simulink model "IEEE30_case"  (R2024b)
settings: Solver=FixedStepAuto  StartTime=0  StopTime=5  FixedStep=1e-7  RelTol=1e-3
values from neighbouring files (symbols this model uses):
  GFL_DFIG_7_C_bus = 0.08    [IEEE30_case_parameters.m]
  GFL_DFIG_7_D_mutual = 2.500000e+3    (= 2500)    [IEEE30_case_parameters.m]
  GFL_DFIG_7_f0 = 60    [IEEE30_case_parameters.m]
  GFL_DFIG_7_gPLLi = 3200    [IEEE30_case_parameters.m]
  GFL_DFIG_7_gPLLp = 650    [IEEE30_case_parameters.m]
  GFL_DFIG_7_H_WT = 0.4    [IEEE30_case_parameters.m]
  GFL_DFIG_7_Hg = 0.8    [IEEE30_case_parameters.m]
  GFL_DFIG_7_Igq_ref = 0    [IEEE30_case_parameters.m]
  GFL_DFIG_7_Ird_ref = 704.45696    [IEEE30_case_parameters.m]
  GFL_DFIG_7_KI_V = -300000    [IEEE30_case_parameters.m]
  GFL_DFIG_7_KP_V = -1000    [IEEE30_case_parameters.m]
  GFL_DFIG_7_Ksh = 1.254300e+4    (= 12543)    [IEEE30_case_parameters.m]
  GFL_DFIG_7_Lg = 0.000483    [IEEE30_case_parameters.m]
  GFL_DFIG_7_Lm_pu = 4    [IEEE30_case_parameters.m]
  GFL_DFIG_7_N = 100    [IEEE30_case_parameters.m]
  GFL_DFIG_7_p = 2    [IEEE30_case_parameters.m]
  GFL_DFIG_7_Pitch = 0    [IEEE30_case_parameters.m]
  GFL_DFIG_7_R = 44    [IEEE30_case_parameters.m]
  GFL_DFIG_7_Rg = 2.000000e-5    (= 2e-05)    [IEEE30_case_parameters.m]
  GFL_DFIG_7_rho = 1.225    [IEEE30_case_parameters.m]
  GFL_DFIG_7_rPLLi = 4500    [IEEE30_case_parameters.m]
  GFL_DFIG_7_rPLLp = 620    [IEEE30_case_parameters.m]
  GFL_DFIG_7_Rs_pu = 0.011    [IEEE30_case_parameters.m]
  GFL_DFIG_7_Sbase = 2.000000e+6    (= 2000000)    [IEEE30_case_parameters.m]
  GFL_DFIG_7_ugq_ref = 0    [IEEE30_case_parameters.m]
  GFL_DFIG_7_usd_ref = 0    [IEEE30_case_parameters.m]
  GFL_DFIG_7_Vbase = 690    [IEEE30_case_parameters.m]
  GFL_DFIG_7_Vdc_ref = 1200    [IEEE30_case_parameters.m]
  GFL_DFIG_7_wind = 12    [IEEE30_case_parameters.m]
  GFL_DFIG_7_wm_ref = 518.184209    [IEEE30_case_parameters.m]
  SG_D_13_D = 0.01056    [IEEE30_case_parameters.m]
  SG_D_13_EnableSaturation = 0    [IEEE30_case_parameters.m]
  SG_D_13_f0 = 60    [IEEE30_case_parameters.m]
  SG_D_13_H = 7.5    [IEEE30_case_parameters.m]
  SG_D_13_K_A = 20    [IEEE30_case_parameters.m]
  SG_D_13_K_E = 1.000000e+1    (= 10)    [IEEE30_case_parameters.m]
  SG_D_13_K_F = 2.363    [IEEE30_case_parameters.m]
  SG_D_13_K_s = 0.5    [IEEE30_case_parameters.m]
  SG_D_13_R_a = 0.001088    [IEEE30_case_parameters.m]
  SG_D_13_S_A = 1    [IEEE30_case_parameters.m]
  SG_D_13_S_B = 0.103    [IEEE30_case_parameters.m]
  SG_D_13_S_N = 10.659857    [IEEE30_case_parameters.m]
  SG_D_13_SpeedPara = 200    [IEEE30_case_parameters.m]
  SG_D_13_T_0 = 0.370163    [IEEE30_case_parameters.m]
  SG_D_13_T_1 = 0.3    [IEEE30_case_parameters.m]
  SG_D_13_T_2 = 0.05    [IEEE30_case_parameters.m]
  SG_D_13_T_3 = 0.02    [IEEE30_case_parameters.m]
  SG_D_13_T_4 = 0.005    [IEEE30_case_parameters.m]
  SG_D_13_T_A = 0.02    [IEEE30_case_parameters.m]
  SG_D_13_T_dd = 8.000000e+0    (= 8)    [IEEE30_case_parameters.m]
  SG_D_13_T_ddd = 0.04    [IEEE30_case_parameters.m]
  SG_D_13_T_E = 0.314    [IEEE30_case_parameters.m]
  SG_D_13_T_F = 0.35    [IEEE30_case_parameters.m]
  SG_D_13_T_qd = 0.8    [IEEE30_case_parameters.m]
  SG_D_13_T_qdd = 0.02    [IEEE30_case_parameters.m]
  SG_D_13_T_speed = 0.1    [IEEE30_case_parameters.m]
  SG_D_13_T_w = 0.5    [IEEE30_case_parameters.m]
  SG_D_13_V_ref = 1.696619    [IEEE30_case_parameters.m]
  SG_D_13_w_ref = 376.991118    [IEEE30_case_parameters.m]
  SG_D_13_x_d = 1.9    [IEEE30_case_parameters.m]
  SG_D_13_x_dd = 0.302    [IEEE30_case_parameters.m]
  SG_D_13_x_ddd = 0.204    [IEEE30_case_parameters.m]
  SG_D_13_x_l = 0.05    [IEEE30_case_parameters.m]
  SG_D_13_x_q = 1.3    [IEEE30_case_parameters.m]
  SG_D_13_x_qd = 0.5    [IEEE30_case_parameters.m]
  SG_D_13_x_qdd = 0.3    [IEEE30_case_parameters.m]
  SG_D_1_D = 0.01056    [IEEE30_case_parameters.m]
  SG_D_1_EnableSaturation = 0    [IEEE30_case_parameters.m]
  SG_D_1_f0 = 60    [IEEE30_case_parameters.m]
  SG_D_1_H = 7.5    [IEEE30_case_parameters.m]
  SG_D_1_K_A = 20    [IEEE30_case_parameters.m]
  SG_D_1_K_E = 1.000000e+1    (= 10)    [IEEE30_case_parameters.m]
  SG_D_1_K_F = 2.363    [IEEE30_case_parameters.m]
  SG_D_1_K_s = 0.5    [IEEE30_case_parameters.m]
  SG_D_1_R_a = 0.001088    [IEEE30_case_parameters.m]
  SG_D_1_S_A = 1    [IEEE30_case_parameters.m]
  SG_D_1_S_B = 0.103    [IEEE30_case_parameters.m]
  SG_D_1_S_N = 10.659857    [IEEE30_case_parameters.m]
  SG_D_1_SpeedPara = 200    [IEEE30_case_parameters.m]
  SG_D_1_T_0 = 0.259812    [IEEE30_case_parameters.m]
  SG_D_1_T_1 = 0.3    [IEEE30_case_parameters.m]
  SG_D_1_T_2 = 0.05    [IEEE30_case_parameters.m]
  SG_D_1_T_3 = 0.02    [IEEE30_case_parameters.m]
  SG_D_1_T_4 = 0.005    [IEEE30_case_parameters.m]
  SG_D_1_T_A = 0.02    [IEEE30_case_parameters.m]
  SG_D_1_T_dd = 8.000000e+0    (= 8)    [IEEE30_case_parameters.m]
  SG_D_1_T_ddd = 0.04    [IEEE30_case_parameters.m]
  SG_D_1_T_E = 0.314    [IEEE30_case_parameters.m]
  SG_D_1_T_F = 0.35    [IEEE30_case_parameters.m]
  SG_D_1_T_qd = 0.8    [IEEE30_case_parameters.m]
  SG_D_1_T_qdd = 0.02    [IEEE30_case_parameters.m]
  SG_D_1_T_speed = 0.1    [IEEE30_case_parameters.m]
  SG_D_1_T_w = 0.5    [IEEE30_case_parameters.m]
  SG_D_1_V_ref = 1.544107    [IEEE30_case_parameters.m]
  SG_D_1_w_ref = 376.991118    [IEEE30_case_parameters.m]
  SG_D_1_x_d = 1.9    [IEEE30_case_parameters.m]
  SG_D_1_x_dd = 0.302    [IEEE30_case_parameters.m]
  SG_D_1_x_ddd = 0.204    [IEEE30_case_parameters.m]
  SG_D_1_x_l = 0.05    [IEEE30_case_parameters.m]
  SG_D_1_x_q = 1.3    [IEEE30_case_parameters.m]
  SG_D_1_x_qd = 0.5    [IEEE30_case_parameters.m]
  SG_D_1_x_qdd = 0.3    [IEEE30_case_parameters.m]
  SG_D_22_D = 0.01056    [IEEE30_case_parameters.m]
  SG_D_22_EnableSaturation = 0    [IEEE30_case_parameters.m]
  SG_D_22_f0 = 60    [IEEE30_case_parameters.m]
  SG_D_22_H = 7.5    [IEEE30_case_parameters.m]
  SG_D_22_K_A = 20    [IEEE30_case_parameters.m]
  SG_D_22_K_E = 1.000000e+1    (= 10)    [IEEE30_case_parameters.m]
  SG_D_22_K_F = 2.363    [IEEE30_case_parameters.m]
  SG_D_22_K_s = 0.5    [IEEE30_case_parameters.m]
  SG_D_22_R_a = 0.001088    [IEEE30_case_parameters.m]
  SG_D_22_S_A = 1    [IEEE30_case_parameters.m]
  SG_D_22_S_B = 0.103    [IEEE30_case_parameters.m]
  SG_D_22_S_N = 10.659857    [IEEE30_case_parameters.m]
  SG_D_22_SpeedPara = 200    [IEEE30_case_parameters.m]
  SG_D_22_T_0 = 0.216121    [IEEE30_case_parameters.m]
  SG_D_22_T_1 = 0.3    [IEEE30_case_parameters.m]
  SG_D_22_T_2 = 0.05    [IEEE30_case_parameters.m]
  SG_D_22_T_3 = 0.02    [IEEE30_case_parameters.m]
  SG_D_22_T_4 = 0.005    [IEEE30_case_parameters.m]
  ... (+126 more)
(part 20 of 27)

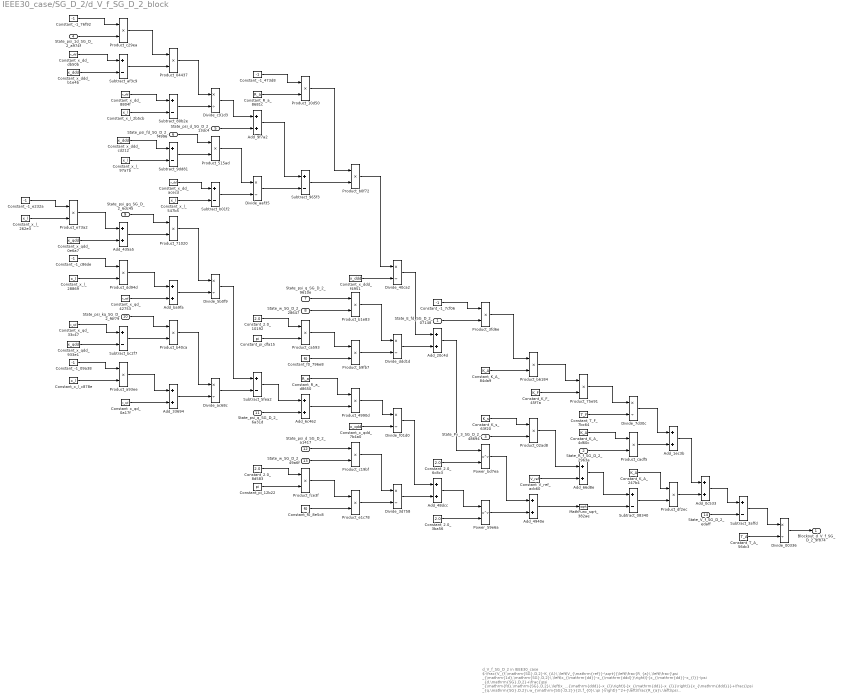
== system IEEE30_case/SG_D_2/d_V_f_SG_D_2_block ==
  note: d_V_f_SG_D_2 in IEEE30_case
      | $-\frac{V_{f,\mathrm{SG},D,2}-K_{A}\,\left(V_{\mathrm{ref}}-\sqrt{{\left(\frac{R_{a}\,\left(\frac{\psi _{\mathrm{1d},\mathrm{SG},D,2}\,\left(x_{\mathrm{dd}}-x_{\mathrm{ddd}}\right)}{x_{\mathrm{dd}}-x_{l}}-\psi _{d,\mathrm{SG},D,2}+\frac{\psi _{\mathrm{fd},\mathrm{SG},D,2}\,\left(x_{\mathrm{ddd}}-x_{l}\right)}{x_{\mathrm{dd}}-x_{l}}\right)}{x_{\mathrm{ddd}}}+\frac{\psi _{q,\mathrm{SG},D,2}\,w_{\mathrm{SG},D,2}}{2\,f_{0}\,\pi }\right)}^2+{\left(\frac{R_{a}\,\left(\psi _{q,\mathrm{SG},D,2}+\frac{\psi _{\mathrm{gq},\mathrm{SG},D,2}\,\left(x_{l}-x_{\mathrm{qdd}}\right)}{x_{l}-x_{\mathrm{qd}}}+\frac{\psi _{\mathrm{kq},\mathrm{SG},D,2}\,\left(x_{\mathrm{qd}}-x_{\mathrm{qdd}}\right)}{x_{l}-x_{\mathrm{qd}}}\right)}{x_{\mathrm{qdd}}}+\frac{\psi _{d,\mathrm{SG},D,2}\,w_{\mathrm{SG},D,2}}{2\,f_{0}\,\pi }\right)}^2}+K_{s}\,\mathrm{Px}_{3,\mathrm{SG},D,2}\right)-K_{A}\,R_{f,\mathrm{SG},D,2}+\frac{E_{\mathrm{fd},\mathrm{SG},D,2}\,K_{A}\,K_{F}}{T_{F}}}{T_{A}}$
      | Automatically generated on 2025-11-01 18:31:41 .
  State_E_fd_SG_D_2_07148 : Inport
  State_R_f_SG_D_2_2963a : Inport  Port=2
  State_Px_3_SG_D_2_48694 : Inport  Port=3
  State_psi_1d_SG_D_2_a974f : Inport  Port=4
  State_psi_d_SG_D_2_13dc4 : Inport  Port=5
  State_psi_fd_SG_D_2_f4996 : Inport  Port=6
  State_psi_q_SG_D_2_9610e : Inport  Port=7
  State_w_SG_D_2_28647 : Inport  Port=8
  State_psi_gq_SG_D_2_6dc45 : Inport  Port=9
  State_psi_kq_SG_D_2_f6f79 : Inport  Port=10
  State_psi_q_SG_D_2_6a31d : Inport  Port=11
  State_psi_d_SG_D_2_a1417 : Inport  Port=12
  State_w_SG_D_2_49a6f : Inport  Port=13
  State_V_f_SG_D_2_edaff : Inport  Port=14
  Add_0c533 : Sum
  Add_1ec3b : Sum
  Add_20c4d : Sum
  Add_33694 : Sum
  Add_435a5 : Sum
  Add_48dcc : Sum
  Add_4940e : Sum
  Add_66d8e : Sum
  Add_6c462 : Sum
  Add_9f7a2 : Sum
  Add_ba9fa : Sum
  Constant_-1_09a38 : Constant  Value=-1
  Constant_-1_473d8 : Constant  Value=-1
  Constant_-1_76f92 : Constant  Value=-1
  Constant_-1_7cf06 : Constant  Value=-1
  Constant_-1_c86de : Constant  Value=-1
  Constant_-1_e232a : Constant  Value=-1
  Constant_2.0_10192 : Constant  Value=2.0
  Constant_2.0_3ba56 : Constant  Value=2.0
  Constant_2.0_6c8c3 : Constant  Value=2.0
  Constant_2.0_8d583 : Constant  Value=2.0
  Constant_K_A_247b4 : Constant  Value=K_A
  Constant_K_A_4d60c : Constant  Value=K_A
  Constant_K_A_84da9 : Constant  Value=K_A
  Constant_K_F_45f7a : Constant  Value=K_F
  Constant_K_s_63f20 : Constant  Value=K_s
  Constant_R_a_8681c : Constant  Value=R_a
  Constant_R_a_d8650 : Constant  Value=R_a
  Constant_T_A_56dc3 : Constant  Value=T_A
  Constant_T_F_7bc64 : Constant  Value=T_F
  Constant_V_ref_acb60 : Constant  Value=V_ref
  Constant_f0_796e8 : Constant  Value=f0
  Constant_f0_8e5c8 : Constant  Value=f0
  Constant_pi_12b22 : Constant  Value=pi
  Constant_pi_dfa15 : Constant  Value=pi
  Constant_x_dd_8804f : Constant  Value=x_dd
  Constant_x_dd_acecd : Constant  Value=x_dd
  Constant_x_dd_db50b : Constant  Value=x_dd
  Constant_x_ddd_b1e4b : Constant  Value=x_ddd
  Constant_x_ddd_cd212 : Constant  Value=x_ddd
  Constant_x_ddd_f4951 : Constant  Value=x_ddd
  Constant_x_l_262e3 : Constant  Value=x_l
  Constant_x_l_28869 : Constant  Value=x_l
  Constant_x_l_2b5cb : Constant  Value=x_l
  Constant_x_l_547b5 : Constant  Value=x_l
  Constant_x_l_97a7b : Constant  Value=x_l
  Constant_x_l_c878e : Constant  Value=x_l
  Constant_x_qd_0a17f : Constant  Value=x_qd
  Constant_x_qd_33c47 : Constant  Value=x_qd
  Constant_x_qd_42753 : Constant  Value=x_qd
  Constant_x_qdd_0e6a7 : Constant  Value=x_qdd
  Constant_x_qdd_7b4a0 : Constant  Value=x_qdd
  Constant_x_qdd_933e1 : Constant  Value=x_qdd
  Divide_00336 : Product  Inputs=*/
  Divide_3d758 : Product  Inputs=*/
  Divide_40ca2 : Product  Inputs=*/
  Divide_5b0f9 : Product  Inputs=*/
  Divide_7d30c : Product  Inputs=*/
  Divide_aaf35 : Product  Inputs=*/
  Divide_ac68c : Product  Inputs=*/
  Divide_c91d3 : Product  Inputs=*/
  Divide_ddd1d : Product  Inputs=*/
  Divide_f01d0 : Product  Inputs=*/
  MathFunc_sqrt_382ae : Sqrt
  Power_59e6a : Math  Operator=pow
  Power_bd7ea : Math  Operator=pow
  Product_02ad8 : Product
  Product_04437 : Product
  Product_10d50 : Product
  Product_3fd6e : Product
  Product_4990d : Product
  Product_515ad : Product
  Product_71020 : Product
  Product_75e91 : Product
  Product_a93ee : Product
  Product_b0f72 : Product
  Product_b1e83 : Product
  Product_b40ca : Product
  Product_b6184 : Product
  Product_b9fb7 : Product
  Product_c19bf : Product
  Product_c29ea : Product
  Product_ca593 : Product
  Product_cadf5 : Product
  Product_dd94d : Product
  Product_df2ec : Product
  Product_e1c78 : Product
  Product_e73a2 : Product
  Product_fce3f : Product
  Subtract_08340 : Sum  Inputs=+-
  Subtract_3affd : Sum  Inputs=+-
  Subtract_5fea2 : Sum  Inputs=+-
  Subtract_80b2e : Sum  Inputs=+-
  Subtract_965f3 : Sum  Inputs=+-
  Subtract_9dd81 : Sum  Inputs=+-
  Subtract_af3c9 : Sum  Inputs=+-
  Subtract_b01f2 : Sum  Inputs=+-
  Subtract_bc2f7 : Sum  Inputs=+-
  Blockout_d_V_f_SG_D_2_9f874 : Outport
  wires:
  Constant_-1_76f92/1 -> Product_c29ea/1
  Constant_2.0_10192/1 -> Product_ca593/1
  Constant_-1_e232a/1 -> Product_e73a2/1
  Product_ca593/1 -> Product_b9fb7/1
  Product_e73a2/1 -> Add_435a5/1
  Constant_x_l_c878e/1 -> Product_a93ee/2
  Constant_x_l_262e3/1 -> Product_e73a2/2
  State_psi_1d_SG_D_2_a974f/1 -> Product_c29ea/2
  Constant_x_l_547b5/1 -> Subtract_b01f2/2
  Constant_x_dd_db50b/1 -> Subtract_af3c9/1
  Product_4990d/1 -> Divide_f01d0/1
  Constant_x_ddd_b1e4b/1 -> Subtract_af3c9/2
  Constant_x_qd_0a17f/1 -> Add_33694/2
  Add_435a5/1 -> Product_71020/2
  Constant_x_qdd_0e6a7/1 -> Add_435a5/2
  Constant_-1_c86de/1 -> Product_dd94d/1
  Constant_x_dd_acecd/1 -> Subtract_b01f2/1
  Subtract_5fea2/1 -> Add_6c462/1
  Power_bd7ea/1 -> Add_4940e/1
  Constant_x_l_28869/1 -> Product_dd94d/2
  Constant_2.0_8d583/1 -> Product_fce3f/1
  Constant_x_qd_33c47/1 -> Subtract_bc2f7/1
  Constant_pi_12b22/1 -> Product_fce3f/2
  Subtract_965f3/1 -> Product_b0f72/2
  Constant_x_qdd_933e1/1 -> Subtract_bc2f7/2
  State_psi_fd_SG_D_2_f4996/1 -> Product_515ad/1
  Constant_-1_09a38/1 -> Product_a93ee/1
  Product_c29ea/1 -> Product_04437/1
  State_w_SG_D_2_49a6f/1 -> Product_c19bf/2
  Subtract_af3c9/1 -> Product_04437/2
  Constant_x_dd_8804f/1 -> Subtract_80b2e/1
  State_psi_q_SG_D_2_6a31d/1 -> Add_6c462/2
  State_w_SG_D_2_28647/1 -> Product_b1e83/2
  Subtract_9dd81/1 -> Product_515ad/2
  Constant_x_l_2b5cb/1 -> Subtract_80b2e/2
  Add_1ec3b/1 -> Add_0c533/1
  Constant_x_ddd_cd212/1 -> Subtract_9dd81/1
  Constant_x_l_97a7b/1 -> Subtract_9dd81/2
  State_psi_gq_SG_D_2_6dc45/1 -> Product_71020/1
  Product_dd94d/1 -> Add_ba9fa/1
  Subtract_b01f2/1 -> Divide_aaf35/2
  Constant_x_qd_42753/1 -> Add_ba9fa/2
  Product_b1e83/1 -> Divide_ddd1d/1
  State_psi_kq_SG_D_2_f6f79/1 -> Product_b40ca/1
  Subtract_bc2f7/1 -> Product_b40ca/2
  Product_515ad/1 -> Divide_aaf35/1
  State_V_f_SG_D_2_edaff/1 -> Subtract_3affd/2
  Product_a93ee/1 -> Add_33694/1
  Product_04437/1 -> Divide_c91d3/1
  Divide_5b0f9/1 -> Subtract_5fea2/1
  Subtract_80b2e/1 -> Divide_c91d3/2
  Product_71020/1 -> Divide_5b0f9/1
  Add_ba9fa/1 -> Divide_5b0f9/2
  Product_b40ca/1 -> Divide_ac68c/1
  Divide_aaf35/1 -> Subtract_965f3/2
  Constant_f0_796e8/1 -> Product_b9fb7/2
  Add_33694/1 -> Divide_ac68c/2
  Divide_c91d3/1 -> Add_9f7a2/1
  State_psi_d_SG_D_2_13dc4/1 -> Add_9f7a2/2
  Divide_ac68c/1 -> Subtract_5fea2/2
  Constant_-1_473d8/1 -> Product_10d50/1
  Constant_R_a_8681c/1 -> Product_10d50/2
  Constant_f0_8e5c8/1 -> Product_e1c78/2
  Add_9f7a2/1 -> Subtract_965f3/1
  Product_10d50/1 -> Product_b0f72/1
  Constant_pi_dfa15/1 -> Product_ca593/2
  State_psi_q_SG_D_2_9610e/1 -> Product_b1e83/1
  Constant_R_a_d8650/1 -> Product_4990d/1
  State_E_fd_SG_D_2_07148/1 -> Product_3fd6e/2
  Add_6c462/1 -> Product_4990d/2
  State_psi_d_SG_D_2_a1417/1 -> Product_c19bf/1
  Product_fce3f/1 -> Product_e1c78/1
  Product_b0f72/1 -> Divide_40ca2/1
  Constant_x_ddd_f4951/1 -> Divide_40ca2/2
  Product_b9fb7/1 -> Divide_ddd1d/2
  Constant_x_qdd_7b4a0/1 -> Divide_f01d0/2
  Product_c19bf/1 -> Divide_3d758/1
  Product_e1c78/1 -> Divide_3d758/2
  Divide_40ca2/1 -> Add_20c4d/1
  Divide_ddd1d/1 -> Add_20c4d/2
  Divide_f01d0/1 -> Add_48dcc/1
  Divide_3d758/1 -> Add_48dcc/2
  Constant_-1_7cf06/1 -> Product_3fd6e/1
  Add_20c4d/1 -> Power_bd7ea/1
  Constant_2.0_6c8c3/1 -> Power_bd7ea/2
  Add_48dcc/1 -> Power_59e6a/1
  Constant_2.0_3ba56/1 -> Power_59e6a/2
  Product_3fd6e/1 -> Product_b6184/1
  Constant_K_A_84da9/1 -> Product_b6184/2
  Constant_K_s_63f20/1 -> Product_02ad8/1
  State_Px_3_SG_D_2_48694/1 -> Product_02ad8/2
  Power_59e6a/1 -> Add_4940e/2
  Product_b6184/1 -> Product_75e91/1
  Constant_K_F_45f7a/1 -> Product_75e91/2
  Product_02ad8/1 -> Add_66d8e/1
  Constant_V_ref_acb60/1 -> Add_66d8e/2
  Add_4940e/1 -> MathFunc_sqrt_382ae/1
  Product_75e91/1 -> Divide_7d30c/1
  Constant_T_F_7bc64/1 -> Divide_7d30c/2
  Constant_K_A_4d60c/1 -> Product_cadf5/1
  State_R_f_SG_D_2_2963a/1 -> Product_cadf5/2
  Add_66d8e/1 -> Subtract_08340/1
  MathFunc_sqrt_382ae/1 -> Subtract_08340/2
  Divide_7d30c/1 -> Add_1ec3b/1
  Product_cadf5/1 -> Add_1ec3b/2
  Constant_K_A_247b4/1 -> Product_df2ec/1
  Subtract_08340/1 -> Product_df2ec/2
  Product_df2ec/1 -> Add_0c533/2
  Add_0c533/1 -> Subtract_3affd/1
  Subtract_3affd/1 -> Divide_00336/1
  Constant_T_A_56dc3/1 -> Divide_00336/2
  Divide_00336/1 -> Blockout_d_V_f_SG_D_2_9f874/1

== system IEEE30_case/SG_D_2/d_psi_1d_SG_D_2_block ==
  note: d_psi_1d_SG_D_2 in IEEE30_case
      | $-\frac{\psi _{\mathrm{1d},\mathrm{SG},D,2}-\psi _{\mathrm{fd},\mathrm{SG},D,2}+\frac{\left(x_{\mathrm{dd}}-x_{l}\right)\,\left(\frac{\psi _{\mathrm{1d},\mathrm{SG},D,2}\,\left(x_{\mathrm{dd}}-x_{\mathrm{ddd}}\right)}{x_{\mathrm{dd}}-x_{l}}-\psi _{d,\mathrm{SG},D,2}+\frac{\psi _{\mathrm{fd},\mathrm{SG},D,2}\,\left(x_{\mathrm{ddd}}-x_{l}\right)}{x_{\mathrm{dd}}-x_{l}}\right)}{x_{\mathrm{ddd}}}}{T_{\mathrm{ddd}}}$
      | Automatically generated on 2025-11-01 18:31:17 .
  State_psi_1d_SG_D_2_46e59 : Inport
  State_psi_fd_SG_D_2_4eec5 : Inport  Port=2
  State_psi_1d_SG_D_2_ea3e5 : Inport  Port=3
  State_psi_d_SG_D_2_140c5 : Inport  Port=4
  State_psi_fd_SG_D_2_f6724 : Inport  Port=5
  Add_553a5 : Sum
  Add_8b957 : Sum
  Add_a40bf : Sum
  Constant_-1_36965 : Constant  Value=-1
  Constant_-1_77d61 : Constant  Value=-1
  Constant_T_ddd_11beb : Constant  Value=T_ddd
  Constant_x_dd_1d866 : Constant  Value=x_dd
  Constant_x_dd_46c81 : Constant  Value=x_dd
  Constant_x_dd_4adc0 : Constant  Value=x_dd
  Constant_x_dd_868cb : Constant  Value=x_dd
  Constant_x_ddd_81e13 : Constant  Value=x_ddd
  Constant_x_ddd_8ebd4 : Constant  Value=x_ddd
  Constant_x_ddd_f80a5 : Constant  Value=x_ddd
  Constant_x_l_73925 : Constant  Value=x_l
  Constant_x_l_aa17b : Constant  Value=x_l
  Constant_x_l_cdd04 : Constant  Value=x_l
  Constant_x_l_d246a : Constant  Value=x_l
  Divide_32af8 : Product  Inputs=*/
  Divide_42413 : Product  Inputs=*/
  Divide_64a93 : Product  Inputs=*/
  Divide_c8e3e : Product  Inputs=*/
  Product_0e046 : Product
  Product_23d08 : Product
  Product_618ac : Product
  Product_95b08 : Product
  Product_a66c9 : Product
  Subtract_03fe7 : Sum  Inputs=+-
  Subtract_29157 : Sum  Inputs=+-
  Subtract_63c3a : Sum  Inputs=+-
  Subtract_6d926 : Sum  Inputs=+-
  Subtract_cffb0 : Sum  Inputs=+-
  Subtract_e3072 : Sum  Inputs=+-
  Blockout_d_psi_1d_SG_D_2_b4ac5 : Outport
  wires:
  Subtract_e3072/1 -> Product_23d08/2
  Constant_x_l_aa17b/1 -> Subtract_03fe7/2
  Divide_32af8/1 -> Add_553a5/2
  Subtract_cffb0/1 -> Product_0e046/2
  Constant_-1_36965/1 -> Product_618ac/1
  Constant_x_dd_4adc0/1 -> Subtract_63c3a/1
  Divide_42413/1 -> Blockout_d_psi_1d_SG_D_2_b4ac5/1
  State_psi_fd_SG_D_2_4eec5/1 -> Add_a40bf/2
  State_psi_1d_SG_D_2_ea3e5/1 -> Product_618ac/2
  Divide_64a93/1 -> Subtract_cffb0/2
  Constant_x_ddd_f80a5/1 -> Subtract_63c3a/2
  State_psi_1d_SG_D_2_46e59/1 -> Product_95b08/2
  Product_618ac/1 -> Product_a66c9/1
  Subtract_63c3a/1 -> Product_a66c9/2
  Constant_x_dd_1d866/1 -> Subtract_03fe7/1
  Constant_x_ddd_8ebd4/1 -> Subtract_e3072/1
  Constant_x_l_73925/1 -> Subtract_e3072/2
  Product_a66c9/1 -> Divide_c8e3e/1
  Subtract_03fe7/1 -> Divide_c8e3e/2
  State_psi_fd_SG_D_2_f6724/1 -> Product_23d08/1
  Constant_x_dd_868cb/1 -> Subtract_6d926/1
  Constant_x_l_cdd04/1 -> Subtract_29157/2
  Constant_x_l_d246a/1 -> Subtract_6d926/2
  Constant_x_ddd_81e13/1 -> Divide_32af8/2
  Divide_c8e3e/1 -> Add_8b957/1
  State_psi_d_SG_D_2_140c5/1 -> Add_8b957/2
  Product_23d08/1 -> Divide_64a93/1
  Subtract_6d926/1 -> Divide_64a93/2
  Constant_x_dd_46c81/1 -> Subtract_29157/1
  Add_8b957/1 -> Subtract_cffb0/1
  Constant_-1_77d61/1 -> Product_95b08/1
  Subtract_29157/1 -> Product_0e046/1
  Product_95b08/1 -> Add_a40bf/1
  Product_0e046/1 -> Divide_32af8/1
  Add_a40bf/1 -> Add_553a5/1
  Add_553a5/1 -> Divide_42413/1
  Constant_T_ddd_11beb/1 -> Divide_42413/2

== system IEEE30_case/SG_D_2/d_psi_d_SG_D_2_block ==
  note: d_psi_d_SG_D_2 in IEEE30_case
      | $2\,\pi \,f_{0}\,\left(v_{d,\mathrm{SG},D,2}\,\sin\left(\theta _{\mathrm{SG},D,2}\right)-v_{q,\mathrm{SG},D,2}\,\cos\left(\theta _{\mathrm{SG},D,2}\right)+\frac{R_{a}\,\left(\frac{\psi _{\mathrm{1d},\mathrm{SG},D,2}\,\left(x_{\mathrm{dd}}-x_{\mathrm{ddd}}\right)}{x_{\mathrm{dd}}-x_{l}}-\psi _{d,\mathrm{SG},D,2}+\frac{\psi _{\mathrm{fd},\mathrm{SG},D,2}\,\left(x_{\mathrm{ddd}}-x_{l}\right)}{x_{\mathrm{dd}}-x_{l}}\right)}{x_{\mathrm{ddd}}}+\frac{\psi _{q,\mathrm{SG},D,2}\,w_{\mathrm{SG},D,2}}{2\,f_{0}\,\pi }\right)$
      | Automatically generated on 2025-11-01 18:31:08 .
  State_psi_1d_SG_D_2_df2dd : Inport
  State_psi_d_SG_D_2_ba6c1 : Inport  Port=2
  State_psi_fd_SG_D_2_fffbd : Inport  Port=3
  Input_v_d_SG_D_2_98b6e : Inport  Port=4
  State_theta_SG_D_2_7fad9 : Inport  Port=5
  Input_v_q_SG_D_2_5c158 : Inport  Port=6
  State_theta_SG_D_2_809cf : Inport  Port=7
  State_psi_q_SG_D_2_54436 : Inport  Port=8
  State_w_SG_D_2_cc748 : Inport  Port=9
  Add_1ebfb : Sum
  Add_63b69 : Sum
  Constant_-1_6ca0d : Constant  Value=-1
  Constant_-2.0_1409b : Constant  Value=-2.0
  Constant_2.0_42c51 : Constant  Value=2.0
  Constant_R_a_27fa6 : Constant  Value=R_a
  Constant_f0_e3338 : Constant  Value=f0
  Constant_f0_fe94e : Constant  Value=f0
  Constant_pi_10ecf : Constant  Value=pi
  Constant_pi_7c0b2 : Constant  Value=pi
  Constant_x_dd_40591 : Constant  Value=x_dd
  Constant_x_dd_65ac5 : Constant  Value=x_dd
  Constant_x_dd_baf94 : Constant  Value=x_dd
  Constant_x_ddd_851e3 : Constant  Value=x_ddd
  Constant_x_ddd_9effc : Constant  Value=x_ddd
  Constant_x_ddd_e26ca : Constant  Value=x_ddd
  Constant_x_l_218e2 : Constant  Value=x_l
  Constant_x_l_5b573 : Constant  Value=x_l
  Constant_x_l_a44df : Constant  Value=x_l
  Divide_3ccb0 : Product  Inputs=*/
  Divide_63f9c : Product  Inputs=*/
  Divide_da75d : Product  Inputs=*/
  Divide_eead1 : Product  Inputs=*/
  MathFunc_cos_24ad6 : Trigonometry  Operator=cos
  MathFunc_sin_91f42 : Trigonometry
  Product_{14361,44426,62010,96773} (4 alike) : Product
  Product_1e194 : Product
  Product_354a5 : Product
  Product_48a05 : Product
  Product_8d88e : Product
  Product_9a8ec : Product
  Product_ae1ce : Product
  Product_ceee8 : Product
  Product_df34b : Product
  Subtract_14ae4 : Sum  Inputs=+-
  Subtract_3cd6b : Sum  Inputs=+-
  Subtract_5791b : Sum  Inputs=+-
  Subtract_85476 : Sum  Inputs=+-
  Subtract_9bf38 : Sum  Inputs=+-
  Subtract_cd5d1 : Sum  Inputs=+-
  Subtract_f9f89 : Sum  Inputs=+-
  Blockout_d_psi_d_SG_D_2_e4800 : Outport
  wires:
  MathFunc_sin_91f42/1 -> Product_df34b/2
  Constant_x_dd_40591/1 -> Subtract_9bf38/1
  Constant_-1_6ca0d/1 -> Product_ae1ce/1
  Constant_x_l_5b573/1 -> Subtract_9bf38/2
  State_psi_1d_SG_D_2_df2dd/1 -> Product_ae1ce/2
  Constant_f0_fe94e/1 -> Product_48a05/2
  Constant_2.0_42c51/1 -> Product_14361/1
  Constant_x_l_218e2/1 -> Subtract_5791b/2
  Constant_x_dd_65ac5/1 -> Subtract_3cd6b/1
  Product_8d88e/1 -> Blockout_d_psi_d_SG_D_2_e4800/1
  Constant_pi_10ecf/1 -> Product_14361/2
  Constant_x_ddd_9effc/1 -> Subtract_3cd6b/2
  Subtract_85476/1 -> Product_8d88e/2
  Product_ae1ce/1 -> Product_9a8ec/1
  Product_14361/1 -> Product_1e194/1
  Subtract_3cd6b/1 -> Product_9a8ec/2
  Divide_eead1/1 -> Subtract_85476/2
  Constant_x_ddd_e26ca/1 -> Subtract_cd5d1/1
  Constant_x_l_a44df/1 -> Subtract_cd5d1/2
  Product_9a8ec/1 -> Divide_3ccb0/1
  Subtract_f9f89/1 -> Add_1ebfb/1
  Subtract_9bf38/1 -> Divide_3ccb0/2
  State_psi_fd_SG_D_2_fffbd/1 -> Product_44426/1
  Subtract_cd5d1/1 -> Product_44426/2
  Constant_x_dd_baf94/1 -> Subtract_5791b/1
  Divide_3ccb0/1 -> Add_63b69/1
  State_psi_d_SG_D_2_ba6c1/1 -> Add_63b69/2
  Product_44426/1 -> Divide_da75d/1
  Subtract_5791b/1 -> Divide_da75d/2
  Add_63b69/1 -> Subtract_14ae4/1
  Divide_da75d/1 -> Subtract_14ae4/2
  Constant_R_a_27fa6/1 -> Product_354a5/1
  Subtract_14ae4/1 -> Product_354a5/2
  Divide_63f9c/1 -> Subtract_f9f89/1
  State_theta_SG_D_2_7fad9/1 -> MathFunc_sin_91f42/1
  Product_354a5/1 -> Divide_63f9c/1
  Constant_-2.0_1409b/1 -> Product_62010/1
  Input_v_d_SG_D_2_98b6e/1 -> Product_df34b/1
  Constant_x_ddd_851e3/1 -> Divide_63f9c/2
  State_theta_SG_D_2_809cf/1 -> MathFunc_cos_24ad6/1
  Product_48a05/1 -> Product_8d88e/1
  Product_df34b/1 -> Subtract_f9f89/2
  Product_62010/1 -> Product_48a05/1
  Input_v_q_SG_D_2_5c158/1 -> Product_ceee8/1
  MathFunc_cos_24ad6/1 -> Product_ceee8/2
  State_psi_q_SG_D_2_54436/1 -> Product_96773/1
  State_w_SG_D_2_cc748/1 -> Product_96773/2
  Constant_f0_e3338/1 -> Product_1e194/2
  Constant_pi_7c0b2/1 -> Product_62010/2
  Product_ceee8/1 -> Add_1ebfb/2
  Product_96773/1 -> Divide_eead1/1
  Product_1e194/1 -> Divide_eead1/2
  Add_1ebfb/1 -> Subtract_85476/1

== system IEEE30_case/SG_D_2/d_psi_fd_SG_D_2_block ==
  note: d_psi_fd_SG_D_2 in IEEE30_case
      | $-\frac{\psi _{\mathrm{fd},\mathrm{SG},D,2}-E_{\mathrm{fd},\mathrm{SG},D,2}+\left(x_{d}-x_{\mathrm{dd}}\right)\,\left(\frac{\frac{\psi _{\mathrm{1d},\mathrm{SG},D,2}\,\left(x_{\mathrm{dd}}-x_{\mathrm{ddd}}\right)}{x_{\mathrm{dd}}-x_{l}}-\psi _{d,\mathrm{SG},D,2}+\frac{\psi _{\mathrm{fd},\mathrm{SG},D,2}\,\left(x_{\mathrm{ddd}}-x_{l}\right)}{x_{\mathrm{dd}}-x_{l}}}{x_{\mathrm{ddd}}}-\frac{\left(x_{\mathrm{dd}}-x_{\mathrm{ddd}}\right)\,\left(\psi _{\mathrm{1d},\mathrm{SG},D,2}-\psi _{\mathrm{fd},\mathrm{SG},D,2}+\frac{\left(x_{\mathrm{dd}}-x_{l}\right)\,\left(\frac{\psi _{\mathrm{1d},\mathrm{SG},D,2}\,\left(x_{\mathrm{dd}}-x_{\mathrm{ddd}}\right)}{x_{\mathrm{dd}}-x_{l}}-\psi _{d,\mathrm{SG},D,2}+\frac{\psi _{\mathrm{fd},\mathrm{SG},D,2}\,\left(x_{\mathrm{ddd}}-x_{l}\right)}{x_{\mathrm{dd}}-x_{l}}\right)}{x_{\mathrm{ddd}}}\right)}{{\left(x_{\mathrm{dd}}-x_{l}\right)}^2}\right)}{T_{\mathrm{dd}}}$
      | Automatically generated on 2025-11-01 18:31:16 .
  State_E_fd_SG_D_2_9e073 : Inport
  State_psi_fd_SG_D_2_a9693 : Inport  Port=2
  State_psi_1d_SG_D_2_36843 : Inport  Port=3
  State_psi_fd_SG_D_2_74282 : Inport  Port=4
  State_psi_1d_SG_D_2_42d8b : Inport  Port=5
  State_psi_d_SG_D_2_4b3f7 : Inport  Port=6
  State_psi_fd_SG_D_2_d0da0 : Inport  Port=7
  State_psi_1d_SG_D_2_a65ff : Inport  Port=8
  State_psi_d_SG_D_2_ea571 : Inport  Port=9
  State_psi_fd_SG_D_2_33a5d : Inport  Port=10
  Add_89e72 : Sum
  Add_bda76 : Sum
  Constant_-1_5d8da : Constant  Value=-1
  Constant_-1_d567e : Constant  Value=-1
  Constant_-1_df985 : Constant  Value=-1
  Constant_2.0_d00af : Constant  Value=2.0
  Constant_T_dd_c33b1 : Constant  Value=T_dd
  Constant_x_d_3bec6 : Constant  Value=x_d
  Constant_x_dd_2654a : Constant  Value=x_dd
  Constant_x_dd_35d89 : Constant  Value=x_dd
  Constant_x_dd_3dab0 : Constant  Value=x_dd
  Constant_x_dd_49b97 : Constant  Value=x_dd
  Constant_x_dd_5107f : Constant  Value=x_dd
  Constant_x_dd_6fcf5 : Constant  Value=x_dd
  Constant_x_dd_b77ee : Constant  Value=x_dd
  Constant_x_dd_ccfa6 : Constant  Value=x_dd
  Constant_x_dd_d0405 : Constant  Value=x_dd
  Constant_x_dd_f5fa7 : Constant  Value=x_dd
  Constant_x_ddd_138bb : Constant  Value=x_ddd
  Constant_x_ddd_2fcd0 : Constant  Value=x_ddd
  Constant_x_ddd_31f43 : Constant  Value=x_ddd
  Constant_x_ddd_38a94 : Constant  Value=x_ddd
  Constant_x_ddd_85702 : Constant  Value=x_ddd
  Constant_x_ddd_be99a : Constant  Value=x_ddd
  Constant_x_ddd_e45f6 : Constant  Value=x_ddd
  Constant_x_l_12728 : Constant  Value=x_l
  Constant_x_l_2384f : Constant  Value=x_l
  Constant_x_l_3369a : Constant  Value=x_l
  Constant_x_l_502c0 : Constant  Value=x_l
  Constant_x_l_8e844 : Constant  Value=x_l
  Constant_x_l_ad53e : Constant  Value=x_l
  Constant_x_l_ba863 : Constant  Value=x_l
  Constant_x_l_c2edc : Constant  Value=x_l
  Divide_12ded : Product  Inputs=*/
  Divide_203f2 : Product  Inputs=*/
  Divide_3c241 : Product  Inputs=*/
  Divide_8473f : Product  Inputs=*/
  Divide_b37b7 : Product  Inputs=*/
  Divide_b90e9 : Product  Inputs=*/
  Divide_f9373 : Product  Inputs=*/
  Divide_fe3e6 : Product  Inputs=*/
  Power_f27f9 : Math  Operator=pow
  Product_19bd0 : Product
  Product_22933 : Product
  Product_53866 : Product
  Product_5c5ca : Product
  Product_7915e : Product
  Product_99b2c : Product
  Product_c0bf3 : Product
  Product_c69e9 : Product
  Product_cdde0 : Product
  Product_f1df4 : Product
  Subtract_04251 : Sum  Inputs=+-
  Subtract_04fdd : Sum  Inputs=+-
  Subtract_07802 : Sum  Inputs=+-
  Subtract_1a333 : Sum  Inputs=+-
  Subtract_1f428 : Sum  Inputs=+-
  Subtract_227c2 : Sum  Inputs=+-
  Subtract_2900f : Sum  Inputs=+-
  Subtract_2c044 : Sum  Inputs=+-
  Subtract_3bae6 : Sum  Inputs=+-
  Subtract_4933a : Sum  Inputs=+-
  Subtract_4a22d : Sum  Inputs=+-
  Subtract_63054 : Sum  Inputs=+-
  Subtract_73adc : Sum  Inputs=+-
  Subtract_7f09d : Sum  Inputs=+-
  Subtract_96f5f : Sum  Inputs=+-
  Subtract_9b979 : Sum  Inputs=+-
  Subtract_9ca98 : Sum  Inputs=+-
  Subtract_bf46b : Sum  Inputs=+-
  Subtract_fe9dc : Sum  Inputs=+-
  Blockout_d_psi_fd_SG_D_2_9f80c : Outport
  wires:
  Constant_x_dd_6fcf5/1 -> Subtract_63054/1
  Constant_-1_5d8da/1 -> Product_cdde0/1
  Constant_x_l_c2edc/1 -> Subtract_07802/2
  Divide_12ded/1 -> Add_bda76/1
  Subtract_04251/1 -> Product_99b2c/2
  Constant_x_l_3369a/1 -> Subtract_63054/2
  Product_99b2c/1 -> Divide_b90e9/1
  State_psi_1d_SG_D_2_42d8b/1 -> Product_cdde0/2
  Constant_x_dd_d0405/1 -> Subtract_73adc/1
  Product_c69e9/1 -> Divide_12ded/1
  Constant_x_dd_49b97/1 -> Subtract_fe9dc/1
  Constant_x_ddd_e45f6/1 -> Subtract_73adc/2
  Constant_x_dd_f5fa7/1 -> Subtract_9ca98/1
  Product_cdde0/1 -> Product_5c5ca/1
  Subtract_73adc/1 -> Product_5c5ca/2
  State_psi_d_SG_D_2_ea571/1 -> Add_bda76/2
  Constant_x_ddd_31f43/1 -> Subtract_04251/1
  Constant_x_l_2384f/1 -> Subtract_04251/2
  Product_5c5ca/1 -> Divide_3c241/1
  Subtract_63054/1 -> Divide_3c241/2
  State_psi_fd_SG_D_2_d0da0/1 -> Product_99b2c/1
  Subtract_2c044/1 -> Product_c0bf3/2
  Constant_x_dd_b77ee/1 -> Subtract_3bae6/1
  Constant_x_l_502c0/1 -> Subtract_3bae6/2
  Product_f1df4/1 -> Product_c0bf3/1
  Divide_3c241/1 -> Add_89e72/1
  State_psi_d_SG_D_2_4b3f7/1 -> Add_89e72/2
  Subtract_3bae6/1 -> Divide_b90e9/2
  Constant_x_dd_2654a/1 -> Subtract_07802/1
  Constant_x_ddd_be99a/1 -> Subtract_2900f/1
  Add_89e72/1 -> Subtract_96f5f/1
  Divide_b90e9/1 -> Subtract_96f5f/2
  Constant_-1_d567e/1 -> Product_19bd0/1
  Product_7915e/1 -> Divide_f9373/1
  State_psi_1d_SG_D_2_a65ff/1 -> Product_19bd0/2
  Subtract_fe9dc/1 -> Product_f1df4/2
  Constant_x_dd_35d89/1 -> Subtract_4a22d/1
  Divide_f9373/1 -> Subtract_9b979/2
  Constant_-1_df985/1 -> Product_f1df4/1
  Constant_x_ddd_138bb/1 -> Subtract_4a22d/2
  Constant_x_ddd_85702/1 -> Divide_203f2/2
  Subtract_07802/1 -> Product_22933/1
  Subtract_96f5f/1 -> Product_22933/2
  State_psi_fd_SG_D_2_74282/1 -> Subtract_227c2/2
  Product_19bd0/1 -> Product_c69e9/1
  Subtract_4a22d/1 -> Product_c69e9/2
  Constant_2.0_d00af/1 -> Power_f27f9/2
  State_psi_1d_SG_D_2_36843/1 -> Subtract_227c2/1
  Constant_x_dd_5107f/1 -> Subtract_04fdd/1
  Subtract_2900f/1 -> Product_7915e/2
  Constant_x_l_12728/1 -> Subtract_04fdd/2
  Constant_x_l_ad53e/1 -> Subtract_2900f/2
  Constant_x_ddd_38a94/1 -> Subtract_fe9dc/2
  Subtract_9ca98/1 -> Divide_f9373/2
  Product_22933/1 -> Divide_203f2/1
  Subtract_04fdd/1 -> Divide_12ded/2
  State_psi_fd_SG_D_2_33a5d/1 -> Product_7915e/1
  Constant_x_l_ba863/1 -> Subtract_9ca98/2
  Constant_x_dd_3dab0/1 -> Subtract_1f428/1
  Subtract_227c2/1 -> Subtract_2c044/1
  Divide_203f2/1 -> Subtract_2c044/2
  Constant_x_l_8e844/1 -> Subtract_1f428/2
  Subtract_1f428/1 -> Power_f27f9/1
  Add_bda76/1 -> Subtract_9b979/1
  Product_c0bf3/1 -> Divide_8473f/1
  Power_f27f9/1 -> Divide_8473f/2
  Subtract_9b979/1 -> Divide_fe3e6/1
  Constant_x_ddd_2fcd0/1 -> Divide_fe3e6/2
  Constant_x_d_3bec6/1 -> Subtract_7f09d/1
  Constant_x_dd_ccfa6/1 -> Subtract_7f09d/2
  Divide_8473f/1 -> Subtract_4933a/1
  Divide_fe3e6/1 -> Subtract_4933a/2
  State_E_fd_SG_D_2_9e073/1 -> Subtract_1a333/1
  State_psi_fd_SG_D_2_a9693/1 -> Subtract_1a333/2
  Subtract_7f09d/1 -> Product_53866/1
  Subtract_4933a/1 -> Product_53866/2
  Subtract_1a333/1 -> Subtract_bf46b/1
  Product_53866/1 -> Subtract_bf46b/2
  Subtract_bf46b/1 -> Divide_b37b7/1
  Constant_T_dd_c33b1/1 -> Divide_b37b7/2
  Divide_b37b7/1 -> Blockout_d_psi_fd_SG_D_2_9f80c/1

== system IEEE30_case/SG_D_2/d_psi_gq_SG_D_2_block ==
  note: d_psi_gq_SG_D_2 in IEEE30_case
      | $-\frac{\psi _{\mathrm{gq},\mathrm{SG},D,2}+\left(x_{q}-x_{\mathrm{qd}}\right)\,\left(\frac{\psi _{q,\mathrm{SG},D,2}+\frac{\psi _{\mathrm{gq},\mathrm{SG},D,2}\,\left(x_{l}-x_{\mathrm{qdd}}\right)}{x_{l}-x_{\mathrm{qd}}}+\frac{\psi _{\mathrm{kq},\mathrm{SG},D,2}\,\left(x_{\mathrm{qd}}-x_{\mathrm{qdd}}\right)}{x_{l}-x_{\mathrm{qd}}}}{x_{\mathrm{qdd}}}+\frac{\left(x_{\mathrm{qd}}-x_{\mathrm{qdd}}\right)\,\left(\psi _{\mathrm{gq},\mathrm{SG},D,2}+\psi _{\mathrm{kq},\mathrm{SG},D,2}+\frac{\left(x_{l}-x_{\mathrm{qd}}\right)\,\left(\psi _{q,\mathrm{SG},D,2}+\frac{\psi _{\mathrm{gq},\mathrm{SG},D,2}\,\left(x_{l}-x_{\mathrm{qdd}}\right)}{x_{l}-x_{\mathrm{qd}}}+\frac{\psi _{\mathrm{kq},\mathrm{SG},D,2}\,\left(x_{\mathrm{qd}}-x_{\mathrm{qdd}}\right)}{x_{l}-x_{\mathrm{qd}}}\right)}{x_{\mathrm{qdd}}}\right)}{{\left(x_{l}-x_{\mathrm{qd}}\right)}^2}\right)}{T_{\mathrm{qd}}}$
      | Automatically generated on 2025-11-01 18:31:22 .
  State_psi_gq_SG_D_2_104a2 : Inport
  State_psi_gq_SG_D_2_afe73 : Inport  Port=2
  State_psi_kq_SG_D_2_5e865 : Inport  Port=3
  State_psi_gq_SG_D_2_1bb75 : Inport  Port=4
  State_psi_kq_SG_D_2_721d7 : Inport  Port=5
  State_psi_q_SG_D_2_83abf : Inport  Port=6
  State_psi_gq_SG_D_2_e51c7 : Inport  Port=7
  State_psi_kq_SG_D_2_7a2a4 : Inport  Port=8
  State_psi_q_SG_D_2_6cd36 : Inport  Port=9
  Add_21c7f : Sum
  Add_2272d : Sum
  Add_3a373 : Sum
  Add_55692 : Sum
  Add_6f089 : Sum
  Add_9a316 : Sum
  Add_c5e13 : Sum
  Add_cff41 : Sum
  Add_d6c76 : Sum
  Add_dab0d : Sum
  Add_f66a3 : Sum
  Add_f8fe5 : Sum
  Constant_-1_10102 : Constant  Value=-1
  Constant_-1_192d4 : Constant  Value=-1
  Constant_-1_290d7 : Constant  Value=-1
  Constant_-1_36899 : Constant  Value=-1
  Constant_-1_3896d : Constant  Value=-1
  Constant_-1_49486 : Constant  Value=-1
  Constant_-1_6c94d : Constant  Value=-1
  Constant_-1_9a49b : Constant  Value=-1
  Constant_-1_c7fce : Constant  Value=-1
  Constant_-1_caba0 : Constant  Value=-1
  Constant_2.0_389d0 : Constant  Value=2.0
  Constant_T_qd_d29d9 : Constant  Value=T_qd
  Constant_x_l_0ae25 : Constant  Value=x_l
  Constant_x_l_12adf : Constant  Value=x_l
  Constant_x_l_1d50c : Constant  Value=x_l
  Constant_x_l_3b729 : Constant  Value=x_l
  Constant_x_l_4b0fb : Constant  Value=x_l
  Constant_x_l_71427 : Constant  Value=x_l
  Constant_x_l_7c493 : Constant  Value=x_l
  Constant_x_l_e27ca : Constant  Value=x_l
  Constant_x_q_d60a7 : Constant  Value=x_q
  Constant_x_qd_2e24b : Constant  Value=x_qd
  Constant_x_qd_30c63 : Constant  Value=x_qd
  Constant_x_qd_320e1 : Constant  Value=x_qd
  Constant_x_qd_3622f : Constant  Value=x_qd
  Constant_x_qd_578ee : Constant  Value=x_qd
  Constant_x_qd_c8aef : Constant  Value=x_qd
  Constant_x_qd_d8f6f : Constant  Value=x_qd
  Constant_x_qd_de86d : Constant  Value=x_qd
  Constant_x_qd_e8870 : Constant  Value=x_qd
  Constant_x_qd_f702b : Constant  Value=x_qd
  Constant_x_qdd_19ca0 : Constant  Value=x_qdd
  Constant_x_qdd_82582 : Constant  Value=x_qdd
  Constant_x_qdd_ac4b7 : Constant  Value=x_qdd
  Constant_x_qdd_b6451 : Constant  Value=x_qdd
  Constant_x_qdd_ba097 : Constant  Value=x_qdd
  Constant_x_qdd_f7649 : Constant  Value=x_qdd
  Constant_x_qdd_fdfde : Constant  Value=x_qdd
  Divide_1c641 : Product  Inputs=*/
  Divide_2a2b0 : Product  Inputs=*/
  Divide_2d9c6 : Product  Inputs=*/
  Divide_2ede0 : Product  Inputs=*/
  Divide_30f9e : Product  Inputs=*/
  Divide_33160 : Product  Inputs=*/
  Divide_60014 : Product  Inputs=*/
  Divide_96e21 : Product  Inputs=*/
  Power_7d008 : Math  Operator=pow
  Product_0c6e7 : Product
  Product_{37177,54883,65103,97917} (4 alike) : Product
  Product_3ed5e : Product
  Product_40b5a : Product
  Product_5283f : Product
  Product_6eed5 : Product
  Product_89c4d : Product
  Product_9a49c : Product
  Product_9d6ad : Product
  Product_b6e50 : Product
  Product_bfbea : Product
  Product_c9315 : Product
  Product_d0ebf : Product
  Product_e22ef : Product
  Subtract_1a0d9 : Sum  Inputs=+-
  Subtract_1ea22 : Sum  Inputs=+-
  Subtract_263b1 : Sum  Inputs=+-
  Subtract_2a63c : Sum  Inputs=+-
  Subtract_4ba7d : Sum  Inputs=+-
  Subtract_9f12a : Sum  Inputs=+-
  Subtract_a0273 : Sum  Inputs=+-
  Subtract_a6d49 : Sum  Inputs=+-
  Blockout_d_psi_gq_SG_D_2_e9d2a : Outport
  wires:
  Constant_x_l_4b0fb/1 -> Product_e22ef/2
  Constant_x_l_3b729/1 -> Product_5283f/2
  Constant_x_qd_de86d/1 -> Subtract_1ea22/1
  Constant_x_l_1d50c/1 -> Product_9d6ad/2
  Constant_x_qdd_ba097/1 -> Subtract_a0273/2
  Constant_-1_10102/1 -> Product_89c4d/1
  Constant_-1_9a49b/1 -> Product_3ed5e/1
  State_psi_gq_SG_D_2_afe73/1 -> Add_3a373/1
  Constant_x_qdd_fdfde/1 -> Subtract_1ea22/2
  Constant_x_qd_e8870/1 -> Subtract_a0273/1
  Constant_x_l_12adf/1 -> Product_89c4d/2
  Constant_x_l_7c493/1 -> Product_3ed5e/2
  Product_89c4d/1 -> Add_dab0d/1
  Product_3ed5e/1 -> Add_2272d/1
  Constant_x_l_71427/1 -> Product_37177/2
  Constant_x_l_0ae25/1 -> Product_0c6e7/2
  Constant_x_qd_f702b/1 -> Add_dab0d/2
  Constant_x_qdd_b6451/1 -> Add_2272d/2
  Constant_-1_c7fce/1 -> Product_37177/1
  Constant_x_qd_3622f/1 -> Add_d6c76/2
  Constant_x_qdd_f7649/1 -> Add_c5e13/2
  State_psi_gq_SG_D_2_1bb75/1 -> Product_d0ebf/1
  Add_dab0d/1 -> Divide_33160/2
  Add_2272d/1 -> Product_d0ebf/2
  Constant_x_qd_320e1/1 -> Subtract_4ba7d/2
  Product_37177/1 -> Add_f66a3/1
  Constant_x_qd_c8aef/1 -> Add_f66a3/2
  State_psi_kq_SG_D_2_721d7/1 -> Product_6eed5/1
  Divide_2a2b0/1 -> Subtract_9f12a/1
  Subtract_1ea22/1 -> Product_6eed5/2
  Product_d0ebf/1 -> Divide_2a2b0/1
  Add_f66a3/1 -> Divide_2a2b0/2
  Add_6f089/1 -> Product_bfbea/2
  Product_6eed5/1 -> Divide_33160/1
  Constant_-1_36899/1 -> Product_0c6e7/1
  Divide_33160/1 -> Subtract_9f12a/2
  Constant_-1_6c94d/1 -> Product_e22ef/1
  Constant_-1_caba0/1 -> Product_5283f/1
  Product_0c6e7/1 -> Add_cff41/1
  Constant_x_qdd_19ca0/1 -> Subtract_1a0d9/2
  Constant_x_qd_d8f6f/1 -> Add_cff41/2
  Subtract_9f12a/1 -> Add_6f089/1
  Constant_-1_192d4/1 -> Product_9d6ad/1
  State_psi_q_SG_D_2_83abf/1 -> Add_6f089/2
  Product_e22ef/1 -> Add_d6c76/1
  Product_5283f/1 -> Add_c5e13/1
  Constant_-1_290d7/1 -> Product_b6e50/1
  Product_bfbea/1 -> Divide_2d9c6/1
  Constant_x_l_e27ca/1 -> Product_b6e50/2
  Product_54883/1 -> Add_9a316/2
  Constant_x_qd_2e24b/1 -> Subtract_1a0d9/1
  Add_cff41/1 -> Product_bfbea/1
  State_psi_gq_SG_D_2_e51c7/1 -> Product_40b5a/1
  Add_d6c76/1 -> Divide_30f9e/2
  Add_c5e13/1 -> Product_40b5a/2
  Product_b6e50/1 -> Add_55692/1
  Constant_x_qd_578ee/1 -> Add_55692/2
  State_psi_kq_SG_D_2_7a2a4/1 -> Product_c9315/1
  Subtract_1a0d9/1 -> Product_c9315/2
  Divide_30f9e/1 -> Subtract_263b1/2
  State_psi_kq_SG_D_2_5e865/1 -> Add_3a373/2
  Product_c9315/1 -> Divide_30f9e/1
  Constant_x_qdd_ac4b7/1 -> Divide_2d9c6/2
  Product_40b5a/1 -> Divide_60014/1
  Add_55692/1 -> Divide_60014/2
  Constant_-1_49486/1 -> Product_97917/1
  Subtract_a0273/1 -> Product_97917/2
  Add_3a373/1 -> Subtract_a6d49/1
  Divide_2d9c6/1 -> Subtract_a6d49/2
  Product_9d6ad/1 -> Add_f8fe5/1
  Constant_x_qd_30c63/1 -> Add_f8fe5/2
  Divide_60014/1 -> Subtract_263b1/1
  Product_97917/1 -> Product_65103/1
  Subtract_a6d49/1 -> Product_65103/2
  Add_f8fe5/1 -> Power_7d008/1
  Constant_2.0_389d0/1 -> Power_7d008/2
  Subtract_263b1/1 -> Add_21c7f/1
  State_psi_q_SG_D_2_6cd36/1 -> Add_21c7f/2
  Product_65103/1 -> Divide_1c641/1
  Power_7d008/1 -> Divide_1c641/2
  Add_21c7f/1 -> Divide_96e21/1
  Constant_x_qdd_82582/1 -> Divide_96e21/2
  Constant_x_q_d60a7/1 -> Subtract_4ba7d/1
  Divide_1c641/1 -> Subtract_2a63c/1
  Divide_96e21/1 -> Subtract_2a63c/2
  Divide_2ede0/1 -> Blockout_d_psi_gq_SG_D_2_e9d2a/1
  Constant_-1_3896d/1 -> Product_9a49c/1
  State_psi_gq_SG_D_2_104a2/1 -> Product_9a49c/2
  Subtract_4ba7d/1 -> Product_54883/1
  Subtract_2a63c/1 -> Product_54883/2
  Product_9a49c/1 -> Add_9a316/1
  Add_9a316/1 -> Divide_2ede0/1
  Constant_T_qd_d29d9/1 -> Divide_2ede0/2

== system IEEE30_case/SG_D_2/d_psi_kq_SG_D_2_block ==
  note: d_psi_kq_SG_D_2 in IEEE30_case
      | $-\frac{\psi _{\mathrm{gq},\mathrm{SG},D,2}+\psi _{\mathrm{kq},\mathrm{SG},D,2}+\frac{\left(x_{l}-x_{\mathrm{qd}}\right)\,\left(\psi _{q,\mathrm{SG},D,2}+\frac{\psi _{\mathrm{gq},\mathrm{SG},D,2}\,\left(x_{l}-x_{\mathrm{qdd}}\right)}{x_{l}-x_{\mathrm{qd}}}+\frac{\psi _{\mathrm{kq},\mathrm{SG},D,2}\,\left(x_{\mathrm{qd}}-x_{\mathrm{qdd}}\right)}{x_{l}-x_{\mathrm{qd}}}\right)}{x_{\mathrm{qdd}}}}{T_{\mathrm{qdd}}}$
      | Automatically generated on 2025-11-01 18:31:25 .
  State_psi_gq_SG_D_2_68a38 : Inport
  State_psi_kq_SG_D_2_4ef7d : Inport  Port=2
  State_psi_gq_SG_D_2_5ea4a : Inport  Port=3
  State_psi_kq_SG_D_2_73d66 : Inport  Port=4
  State_psi_q_SG_D_2_69b92 : Inport  Port=5
  Add_41eda : Sum
  Add_56500 : Sum
  Add_88306 : Sum
  Add_907c2 : Sum
  Add_9f874 : Sum
  Add_f1d29 : Sum
  Constant_-1_0031c : Constant  Value=-1
  Constant_-1_1bbc6 : Constant  Value=-1
  Constant_-1_49c6c : Constant  Value=-1
  Constant_-1_c45d6 : Constant  Value=-1
  Constant_-1_d2115 : Constant  Value=-1
  Constant_T_qdd_cf2dd : Constant  Value=T_qdd
  Constant_x_l_3abd7 : Constant  Value=x_l
  Constant_x_l_889e8 : Constant  Value=x_l
  Constant_x_l_90707 : Constant  Value=x_l
  Constant_x_l_9a825 : Constant  Value=x_l
  Constant_x_qd_7302c : Constant  Value=x_qd
  Constant_x_qd_a1327 : Constant  Value=x_qd
  Constant_x_qd_aa121 : Constant  Value=x_qd
  Constant_x_qd_c3e6d : Constant  Value=x_qd
  Constant_x_qdd_07837 : Constant  Value=x_qdd
  Constant_x_qdd_54d8f : Constant  Value=x_qdd
  Constant_x_qdd_ff2a7 : Constant  Value=x_qdd
  Divide_18b1f : Product  Inputs=*/
  Divide_5686b : Product  Inputs=*/
  Divide_d8f4e : Product  Inputs=*/
  Divide_ffb92 : Product  Inputs=*/
  Product_33be3 : Product
  Product_40274 : Product
  Product_452e2 : Product
  Product_4d14b : Product
  Product_504a8 : Product
  Product_d385a : Product
  Product_ea59d : Product
  Product_f0a41 : Product
  Subtract_1b49b : Sum  Inputs=+-
  Subtract_8fcae : Sum  Inputs=+-
  Subtract_f4fa5 : Sum  Inputs=+-
  Blockout_d_psi_kq_SG_D_2_68567 : Outport
  wires:
  State_psi_kq_SG_D_2_4ef7d/1 -> Subtract_f4fa5/2
  Constant_-1_49c6c/1 -> Product_504a8/1
  Constant_-1_d2115/1 -> Product_d385a/1
  Constant_x_l_90707/1 -> Product_d385a/2
  Constant_x_qdd_07837/1 -> Add_88306/2
  Constant_x_l_9a825/1 -> Product_504a8/2
  Constant_x_qd_c3e6d/1 -> Subtract_1b49b/1
  Constant_T_qdd_cf2dd/1 -> Divide_ffb92/2
  Constant_-1_c45d6/1 -> Product_f0a41/1
  Product_d385a/1 -> Add_88306/1
  Constant_x_qdd_ff2a7/1 -> Subtract_1b49b/2
  Constant_x_l_3abd7/1 -> Product_f0a41/2
  Divide_ffb92/1 -> Blockout_d_psi_kq_SG_D_2_68567/1
  State_psi_gq_SG_D_2_5ea4a/1 -> Product_4d14b/1
  Add_88306/1 -> Product_4d14b/2
  Product_504a8/1 -> Add_41eda/1
  Constant_x_qd_7302c/1 -> Add_41eda/2
  Product_40274/1 -> Divide_5686b/1
  State_psi_kq_SG_D_2_73d66/1 -> Product_33be3/1
  Subtract_1b49b/1 -> Product_33be3/2
  Product_f0a41/1 -> Add_9f874/1
  Constant_x_qd_a1327/1 -> Add_9f874/2
  Product_33be3/1 -> Divide_18b1f/1
  Product_4d14b/1 -> Divide_d8f4e/1
  Add_41eda/1 -> Divide_d8f4e/2
  Add_9f874/1 -> Divide_18b1f/2
  State_psi_q_SG_D_2_69b92/1 -> Add_f1d29/2
  Constant_-1_1bbc6/1 -> Product_452e2/1
  Constant_x_l_889e8/1 -> Product_452e2/2
  Divide_d8f4e/1 -> Subtract_8fcae/1
  Divide_18b1f/1 -> Subtract_8fcae/2
  Product_452e2/1 -> Add_907c2/1
  Constant_x_qd_aa121/1 -> Add_907c2/2
  Subtract_8fcae/1 -> Add_f1d29/1
  Constant_x_qdd_54d8f/1 -> Divide_5686b/2
  Constant_-1_0031c/1 -> Product_ea59d/1
  State_psi_gq_SG_D_2_68a38/1 -> Product_ea59d/2
  Add_907c2/1 -> Product_40274/1
  Add_f1d29/1 -> Product_40274/2
  Product_ea59d/1 -> Subtract_f4fa5/1
  Subtract_f4fa5/1 -> Add_56500/1
  Divide_5686b/1 -> Add_56500/2
  Add_56500/1 -> Divide_ffb92/1

== system IEEE30_case/SG_D_2/d_psi_q_SG_D_2_block ==
  note: d_psi_q_SG_D_2 in IEEE30_case
      | $2\,\pi \,f_{0}\,\left(v_{d,\mathrm{SG},D,2}\,\cos\left(\theta _{\mathrm{SG},D,2}\right)+v_{q,\mathrm{SG},D,2}\,\sin\left(\theta _{\mathrm{SG},D,2}\right)-\frac{R_{a}\,\left(\psi _{q,\mathrm{SG},D,2}+\frac{\psi _{\mathrm{gq},\mathrm{SG},D,2}\,\left(x_{l}-x_{\mathrm{qdd}}\right)}{x_{l}-x_{\mathrm{qd}}}+\frac{\psi _{\mathrm{kq},\mathrm{SG},D,2}\,\left(x_{\mathrm{qd}}-x_{\mathrm{qdd}}\right)}{x_{l}-x_{\mathrm{qd}}}\right)}{x_{\mathrm{qdd}}}-\frac{\psi _{d,\mathrm{SG},D,2}\,w_{\mathrm{SG},D,2}}{2\,f_{0}\,\pi }\right)$
      | Automatically generated on 2025-11-01 18:31:13 .
  State_psi_gq_SG_D_2_77760 : Inport
  State_psi_kq_SG_D_2_d2951 : Inport  Port=2
  State_psi_q_SG_D_2_22b60 : Inport  Port=3
  Input_v_d_SG_D_2_67bf0 : Inport  Port=4
  State_theta_SG_D_2_05bbc : Inport  Port=5
  Input_v_q_SG_D_2_2e6d8 : Inport  Port=6
  State_theta_SG_D_2_018ce : Inport  Port=7
  State_psi_d_SG_D_2_4e236 : Inport  Port=8
  State_w_SG_D_2_5f632 : Inport  Port=9
  Add_1c927 : Sum
  Add_217d8 : Sum
  Add_2628e : Sum
  Add_8e13f : Sum
  Add_ebe31 : Sum
  Constant_-1_1eec3 : Constant  Value=-1
  Constant_-1_3405d : Constant  Value=-1
  Constant_-1_b59c3 : Constant  Value=-1
  Constant_-2.0_40b87 : Constant  Value=-2.0
  Constant_2.0_d24e6 : Constant  Value=2.0
  Constant_R_a_a4ec3 : Constant  Value=R_a
  Constant_f0_42aa5 : Constant  Value=f0
  Constant_f0_8902e : Constant  Value=f0
  Constant_pi_3ae92 : Constant  Value=pi
  Constant_pi_f24c4 : Constant  Value=pi
  Constant_x_l_469e0 : Constant  Value=x_l
  Constant_x_l_779d3 : Constant  Value=x_l
  Constant_x_l_7d43f : Constant  Value=x_l
  Constant_x_qd_023dc : Constant  Value=x_qd
  Constant_x_qd_3f8f6 : Constant  Value=x_qd
  Constant_x_qd_f2f5c : Constant  Value=x_qd
  Constant_x_qdd_002fe : Constant  Value=x_qdd
  Constant_x_qdd_969ae : Constant  Value=x_qdd
  Constant_x_qdd_96cf2 : Constant  Value=x_qdd
  Divide_00829 : Product  Inputs=*/
  Divide_2be33 : Product  Inputs=*/
  Divide_3dcd6 : Product  Inputs=*/
  Divide_4354f : Product  Inputs=*/
  MathFunc_cos_4024a : Trigonometry  Operator=cos
  MathFunc_sin_2aba2 : Trigonometry
  Product_024d3 : Product
  Product_0ff11 : Product
  Product_15629 : Product
  Product_22187 : Product
  Product_3cfba : Product
  Product_487b0 : Product
  Product_582be : Product
  Product_74fee : Product
  Product_89a17 : Product
  Product_9b552 : Product
  Product_9ce74 : Product
  Product_a2705 : Product
  Product_aea2b : Product
  Product_ee081 : Product
  Subtract_1013c : Sum  Inputs=+-
  Subtract_5908a : Sum  Inputs=+-
  Subtract_61671 : Sum  Inputs=+-
  Subtract_926fe : Sum  Inputs=+-
  Blockout_d_psi_q_SG_D_2_4be96 : Outport
  wires:
  Constant_x_qdd_969ae/1 -> Subtract_1013c/2
  Constant_x_l_7d43f/1 -> Product_aea2b/2
  Constant_-1_b59c3/1 -> Product_89a17/1
  Constant_x_l_469e0/1 -> Product_89a17/2
  Product_89a17/1 -> Add_ebe31/1
  Constant_pi_f24c4/1 -> Product_582be/2
  State_psi_gq_SG_D_2_77760/1 -> Product_9ce74/1
  Constant_x_l_779d3/1 -> Product_9b552/2
  State_w_SG_D_2_5f632/1 -> Product_74fee/2
  Constant_x_qd_023dc/1 -> Add_8e13f/2
  Constant_x_qdd_96cf2/1 -> Add_ebe31/2
  Constant_2.0_d24e6/1 -> Product_582be/1
  Constant_-1_3405d/1 -> Product_9b552/1
  Constant_x_qd_f2f5c/1 -> Subtract_1013c/1
  Constant_-1_1eec3/1 -> Product_aea2b/1
  State_psi_q_SG_D_2_22b60/1 -> Add_2628e/2
  Add_ebe31/1 -> Product_9ce74/2
  Product_582be/1 -> Product_0ff11/1
  Product_9b552/1 -> Add_217d8/1
  Constant_pi_3ae92/1 -> Product_22187/2
  Constant_f0_42aa5/1 -> Product_0ff11/2
  Constant_x_qd_3f8f6/1 -> Add_217d8/2
  State_psi_kq_SG_D_2_d2951/1 -> Product_a2705/1
  Subtract_1013c/1 -> Product_a2705/2
  Product_aea2b/1 -> Add_8e13f/1
  Input_v_q_SG_D_2_2e6d8/1 -> Product_024d3/1
  Product_9ce74/1 -> Divide_00829/1
  Product_0ff11/1 -> Divide_4354f/2
  Add_217d8/1 -> Divide_00829/2
  Product_a2705/1 -> Divide_2be33/1
  Add_8e13f/1 -> Divide_2be33/2
  Divide_00829/1 -> Subtract_61671/1
  State_theta_SG_D_2_05bbc/1 -> MathFunc_cos_4024a/1
  Divide_2be33/1 -> Subtract_61671/2
  Subtract_61671/1 -> Add_2628e/1
  MathFunc_cos_4024a/1 -> Product_487b0/2
  Constant_R_a_a4ec3/1 -> Product_15629/1
  Add_2628e/1 -> Product_15629/2
  State_theta_SG_D_2_018ce/1 -> MathFunc_sin_2aba2/1
  Product_15629/1 -> Divide_3dcd6/1
  Product_22187/1 -> Product_3cfba/1
  Product_024d3/1 -> Subtract_926fe/2
  Constant_x_qdd_002fe/1 -> Divide_3dcd6/2
  Input_v_d_SG_D_2_67bf0/1 -> Product_487b0/1
  Add_1c927/1 -> Product_ee081/2
  Divide_3dcd6/1 -> Subtract_5908a/1
  Product_487b0/1 -> Subtract_5908a/2
  MathFunc_sin_2aba2/1 -> Product_024d3/2
  Product_ee081/1 -> Blockout_d_psi_q_SG_D_2_4be96/1
  State_psi_d_SG_D_2_4e236/1 -> Product_74fee/1
  Constant_-2.0_40b87/1 -> Product_22187/1
  Product_3cfba/1 -> Product_ee081/1
  Subtract_5908a/1 -> Subtract_926fe/1
  Product_74fee/1 -> Divide_4354f/1
  Constant_f0_8902e/1 -> Product_3cfba/2
  Subtract_926fe/1 -> Add_1c927/1
  Divide_4354f/1 -> Add_1c927/2

== system IEEE30_case/SG_D_2/d_theta_SG_D_2_block ==
  note: d_theta_SG_D_2 in IEEE30_case
      | $w_{\mathrm{SG},D,2}-2\,\pi \,f_{0}$
      | Automatically generated on 2025-11-01 18:31:32 .
  State_w_SG_D_2_d4d26 : Inport
  Add_a02fc : Sum
  Constant_-2.0_dd3ec : Constant  Value=-2.0
  Constant_f0_98abf : Constant  Value=f0
  Constant_pi_7a596 : Constant  Value=pi
  Product_11c54 : Product
  Product_6af23 : Product
  Blockout_d_theta_SG_D_2_cbd9d : Outport
  wires:
  Constant_-2.0_dd3ec/1 -> Product_11c54/1
  Constant_pi_7a596/1 -> Product_11c54/2
  Add_a02fc/1 -> Blockout_d_theta_SG_D_2_cbd9d/1
  Product_11c54/1 -> Product_6af23/1
  Constant_f0_98abf/1 -> Product_6af23/2
  Product_6af23/1 -> Add_a02fc/1
  State_w_SG_D_2_d4d26/1 -> Add_a02fc/2
